simulink model "LT_PA105"  (R2025b)
settings: Solver=FixedStepAuto  StartTime=0.0  StopTime=inf  FixedStep=1E-3  RelTol=1e-3
libraries: aerolibanimutils x1
settings Model: Creator=abstract  LastModifiedBy=abstract
settings DataIOCC: SaveOutput=off  SignalLogging=off  DSMLogging=off  SaveTime=off  ReturnWorkspaceOutputs=off
settings OptimizationCC: DefaultParameterBehavior=Inlined  EnhancedBackFolding=on  PassReuseOutputArgsAs=Individual arguments  ZeroExternalMemoryAtStartup=off  ZeroInternalMemoryAtStartup=off  OptimizeBlockOrder=speed  DifferentSizesBufferReuse=on  OptimizationCustomize=off  EfficientTunableParamExpr=on
settings DebuggingCC: ParameterTunabilityLossMsg=error
settings SFSimCC: MATLABDynamicMemAlloc=off
settings RTWCC: SystemTargetFile=ert.tlc  GenCodeOnly=on  TemplateMakefile=ert_default_tmf  CustomHeaderCode="#include \"HAL.h\""  Description=Embedded Coder
settings CodeAppCC: ForceParamTrailComments=on  IgnoreCustomStorageClasses=off  OperatorAnnotations=on  SimulinkDataObjDesc=on  SFDataObjDesc=on  InsertBlockDesc=on
settings ERTTargetCC: ERTCustomFileTemplate=example_file_process.tlc  TargetLangStandard=C99 (ISO)  GenerateSampleERTMain=on  SupportNonFinite=off  SupportComplex=off

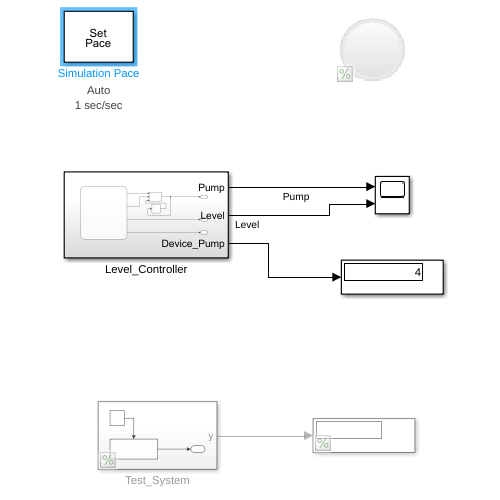
[thumbnail: Simulink's stored preview of the top-level diagram]
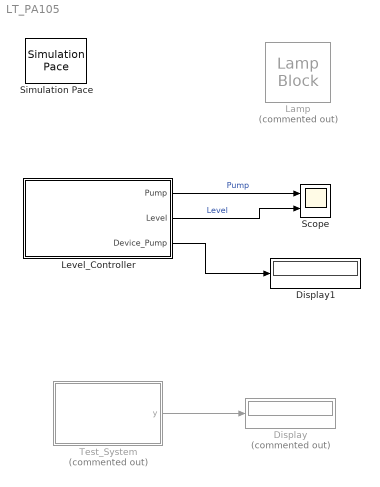
== system LT_PA105 ==
  Display : Display  Commented=on
  Display1 : Display
  Lamp : LampBlock  Commented=on  LabelPosition=Hide  DefaultColor=[192.0, 192.0, 192.0]
  Level_Controller : Subsystem
  Scope : Scope  NumInputPorts=2
      settings: ActiveDisplayYMinimum=-1  ActiveDisplayYMaximum=1
  Simulation Pace : aerolibanimutils/Simulation Pace  SimulationPace=1  SleepMode=Auto  OutputPaceError=off  SampleTime=-1
  Test_System : Subsystem  Commented=on
  wires:
  Test_System/1(y) -> Display/1
  Level_Controller/3(Device_Pump) -> Display1/1
  Level_Controller/1(Pump) -> Scope/1  "Pump"
  Level_Controller/2(Level) -> Scope/2  "Level"

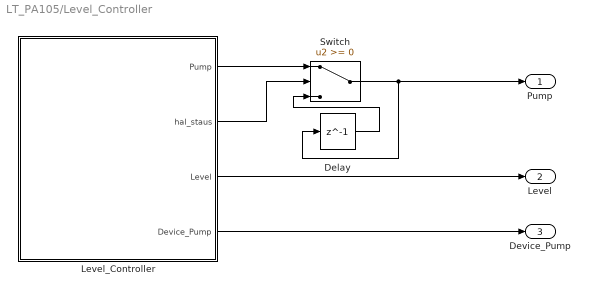
== system LT_PA105/Level_Controller ==
  Delay : Delay  DelayLength=1  InputProcessing=Columns as channels (frame based)
  Level_Controller : Stateflow chart  TreatAsAtomicUnit=on
  Switch : Switch  SaturateOnIntegerOverflow=off  InputSameDT=off
  Pump : Outport
  Level : Outport  Port=2
  Device_Pump : Outport  Port=3
  wires:
  Level_Controller/3(Level) -> Level/1
  Level_Controller/2(hal_staus) -> Switch/2
  Level_Controller/1(Pump) -> Switch/1
  Delay/1 -> Switch/3
  Switch/1 -> Pump/1, Delay/1
  Level_Controller/4(Device_Pump) -> Device_Pump/1

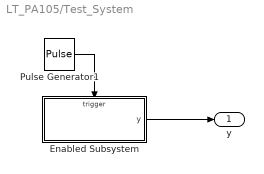
== system LT_PA105/Test_System ==
  Enabled Subsystem : Subsystem  TreatAsAtomicUnit=on
  Pulse Generator1 : DiscretePulseGenerator  PulseType=Time based  Period=1  PulseWidth=5
  y : Outport
  wires:
  Pulse Generator1/1 -> Enabled Subsystem/Trigger
  Enabled Subsystem/1(y) -> y/1

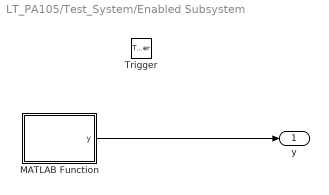
== system LT_PA105/Test_System/Enabled Subsystem ==
  Trigger : TriggerPort  VariantControl=(inherit)  PortDimensions=1
  MATLAB Function : MATLAB Function  TreatAsAtomicUnit=on
  y : Outport
  wires:
  MATLAB Function/1(y) -> y/1

== matlab function LT_PA105/Test_System/Enabled Subsystem/MATLAB Function ==
  data: y output
function y = fcn()

persistent x
if isempty(x)
    x = 0;
end

x = x + 1;

y = x;

== stateflow chart LT_PA105/Level_Controller/Level_Controller ==
  (default) -> (junction 16) : {
      | [hal_staus, level] = LT_PA105_Get_Level();
      | Device_Pump = LT_PA105_Get_Pump();
      | }
  (junction 16) -> (junction 17) [order 1] : [hal_staus == 0]
  (junction 16) -> (junction 18) [order 2] : {Pump = -1;}
  (junction 17) -> (junction 19) : {Level = level;}
  (junction 19) -> (junction 50) [order 1] : [level >= 10]
  (junction 19) -> (junction 54) [order 2] : {Pump = 0;}
  (junction 50) -> (junction 56) : {Pump = 1;}
  (junction 54) -> (junction 18)
  (junction 56) -> (junction 54)
  (junction 18) -> (junction 20)
  data: Pump output single; hal_staus output; level local; Level output; Device_Pump output
